simulink model "Dynamics"  (R2025b)
settings: Solver=VariableStepAuto  StartTime=0.0  StopTime=400000000.0  RelTol=1e-3
values from neighbouring files (symbols this model uses):
  Jc = [400, 0, 0 ... (first row only)    [model.m]
  Jc1 = inv(Jc)    [model.m]
  mu = 3.986004418e14    (= 398600441800000)    [model.m]
  r = 1e6    (= 1000000)    [model.m]
libraries: matrix_library x2, dspmathops x1
settings Model: Creator=sstef  LastModifiedBy=sstef

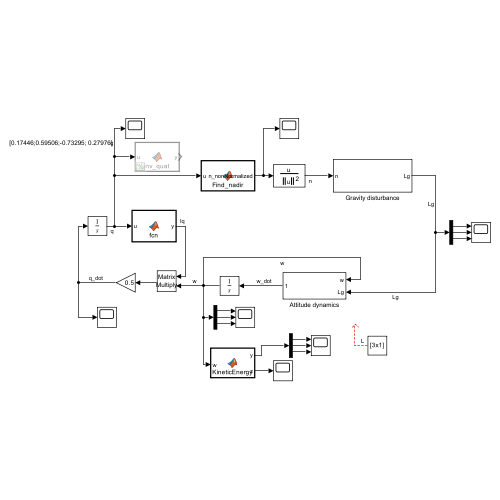
[thumbnail: Simulink's stored preview of the top-level diagram]
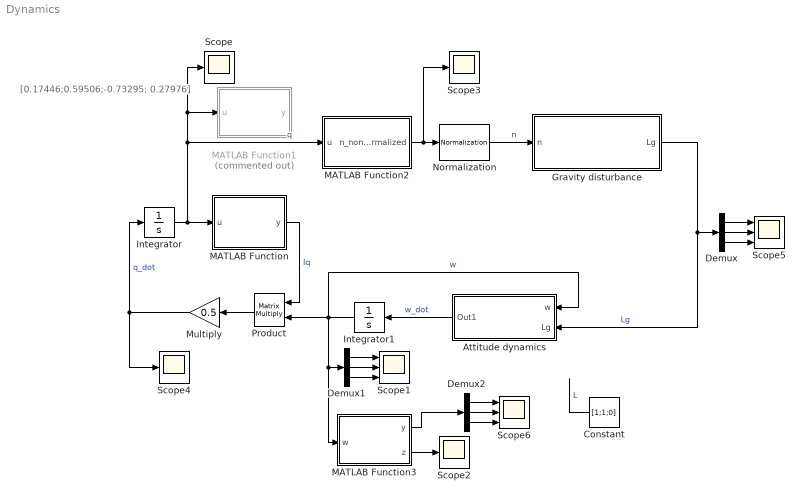
== system Dynamics ==
  note: [0.17446;0.59506;-0.73295; 0.27976]
  Attitude dynamics : Subsystem
  Constant : Constant  Value=[1;1;0]
  Demux : Demux  Outputs=3
  Demux1 : Demux  Outputs=3
  Demux2 : Demux  Outputs=3
  Gravity disturbance : Subsystem
  Integrator : Integrator  InitialCondition=[0.17446;0.59506;-0.73295; 0.27976]  AbsoluteTolerance=0.0001
  Integrator1 : Integrator  AbsoluteTolerance=0.000001
  MATLAB Function : MATLAB Function  TreatAsAtomicUnit=on
  MATLAB Function1 : MATLAB Function  Commented=on  TreatAsAtomicUnit=on
  MATLAB Function2 : MATLAB Function  TreatAsAtomicUnit=on
  MATLAB Function3 : MATLAB Function  TreatAsAtomicUnit=on
  Multiply : Gain  Gain=0.5
  Normalization : dspmathops/Normalization  NormType=Squared 2-norm  Bias=1e-10  NormOver=Each column  Dimension=1  roundingMode=Floor  overflowMode=off  accumDataTypeStr=Inherit: Same as product output  accumLastDataTypeStr=Inherit: Same as product output  outputDataTypeStr=Inherit: Same as product output  outputMin=[]  outputMax=[]  outputLastDataTypeStr=Inherit: Same as product output
  Product : Product  Multiplication=Matrix(*)
  Scope{,2..4} (4 alike) : Scope
      Scope settings: ActiveDisplayYMinimum=-1.1073586484383933  ActiveDisplayYMaximum=1.0833772002903839
      Scope2 settings: ActiveDisplayYMinimum=-0.0045801648053489111  ActiveDisplayYMaximum=0.041221483248140206  DataLoggingVariableName=ScopeData2
      Scope3 settings: ActiveDisplayYMinimum=-1.0201256866840489  ActiveDisplayYMaximum=1.2244583915622078  DataLoggingVariableName=ScopeData6
      Scope4 settings: ActiveDisplayYMinimum=-1.7498948486538512E+34  ActiveDisplayYMaximum=1.6554770346850636E+34  DataLoggingVariableName=ScopeData7
  Scope1 : Scope  NumInputPorts=3
      settings: ActiveDisplayYMinimum=-0.0069359480951209015  ActiveDisplayYMaximum=0.0069181215637571323
  Scope5 : Scope  NumInputPorts=3
      settings: ActiveDisplayYMinimum=-0.013350016010267451  ActiveDisplayYMaximum=0.013181324777865785  DataLoggingVariableName=ScopeData8
  Scope6 : Scope  NumInputPorts=3
      settings: ActiveDisplayYMinimum=-3.5092099871581417  ActiveDisplayYMaximum=3.5511518209448742  DataLoggingVariableName=ScopeData9
  wires:
  Integrator/1 -> MATLAB Function2/1(u), Scope/1, MATLAB Function1/1(u), MATLAB Function/1(u)  "q"
  Product/1 -> Multiply/1
  MATLAB Function/1(y) -> Product/1  "Iq"
  Multiply/1 -> Integrator/1, Scope4/1  "q_dot"
  Integrator1/1 -> Product/2, MATLAB Function3/1(w), Demux1/1, Attitude dynamics/1(w)  "w"
  Attitude dynamics/1(Out1) -> Integrator1/1  "w_dot"
  Constant/1 -> ?  "L"
  MATLAB Function2/1(n_nonNormalized) -> Scope3/1, Normalization/1
  Demux/2 -> Scope5/2
  Demux/3 -> Scope5/3
  Demux/1 -> Scope5/1
  Demux1/1 -> Scope1/1
  Demux1/3 -> Scope1/3
  Demux1/2 -> Scope1/2
  Gravity disturbance/1(Lg) -> Attitude dynamics/2(Lg), Demux/1  "Lg"
  Normalization/1 -> Gravity disturbance/1(n)  "n"
  MATLAB Function3/1(y) -> Demux2/1
  MATLAB Function3/2(z) -> Scope2/1
  Demux2/2 -> Scope6/2
  Demux2/3 -> Scope6/3
  Demux2/1 -> Scope6/1

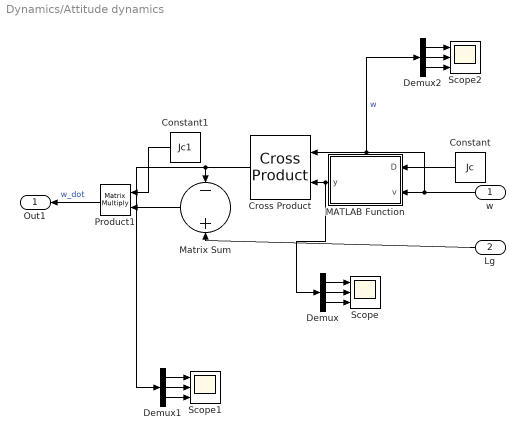
== system Dynamics/Attitude dynamics ==
  w : Inport
  Lg : Inport  Port=2
  Constant : Constant  Value=Jc
  Constant1 : Constant  Value=Jc1
  Cross Product : matrix_library/Cross Product
  Demux : Demux  Outputs=3
  Demux1 : Demux  Outputs=3
  Demux2 : Demux  Outputs=3
  MATLAB Function : MATLAB Function  TreatAsAtomicUnit=on
  Matrix Sum : Sum  Inputs=-+
  Product1 : Product  Multiplication=Matrix(*)
  Scope : Scope  NumInputPorts=3
      settings: ActiveDisplayYMinimum=-84.730783605714521  ActiveDisplayYMaximum=82.344369944838959  DataLoggingVariableName=ScopeData3
  Scope1 : Scope  NumInputPorts=3
      settings: ActiveDisplayYMinimum=-1.8791066376898631E-10  ActiveDisplayYMaximum=4.2850622121844011E-11  DataLoggingVariableName=ScopeData4
  Scope2 : Scope  NumInputPorts=3
      settings: ActiveDisplayYMinimum=-0.0027775205734021252  ActiveDisplayYMaximum=0.024997685160619131  DataLoggingVariableName=ScopeData5
  Out1 : Outport
  wires:
  w/1 -> Demux2/1, Cross Product/1, MATLAB Function/2(v)  "w"
  Lg/1 -> Matrix Sum/2
  Constant1/1 -> Product1/1
  Matrix Sum/1 -> Product1/2
  Product1/1 -> Out1/1  "w_dot"
  Constant/1 -> MATLAB Function/1(D)
  MATLAB Function/1(y) -> Demux/1, Cross Product/2
  Demux/1 -> Scope/1
  Demux/2 -> Scope/2
  Demux/3 -> Scope/3
  Demux1/2 -> Scope1/2
  Demux1/1 -> Scope1/1
  Cross Product/1 -> Demux1/1, Matrix Sum/1
  Demux1/3 -> Scope1/3
  Demux2/2 -> Scope2/2
  Demux2/1 -> Scope2/1
  Demux2/3 -> Scope2/3

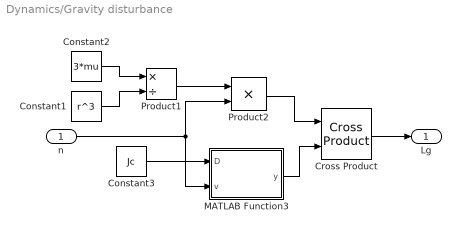
== system Dynamics/Gravity disturbance ==
  n : Inport
  Constant1 : Constant  Value=r^3
  Constant2 : Constant  Value=3*mu
  Constant3 : Constant  Value=Jc
  Cross Product : matrix_library/Cross Product
  MATLAB Function3 : MATLAB Function  TreatAsAtomicUnit=on
  Product1 : Product  Inputs=*/
  Product2 : Product
  Lg : Outport
  wires:
  Cross Product/1 -> Lg/1
  Product1/1 -> Product2/1
  n/1 -> Product2/2, MATLAB Function3/2(v)
  MATLAB Function3/1(y) -> Cross Product/2
  Constant1/1 -> Product1/2
  Constant2/1 -> Product1/1
  Constant3/1 -> MATLAB Function3/1(D)
  Product2/1 -> Cross Product/1

== matlab function Dynamics/MATLAB Function ==
  data: u input size=4 1; y output size=4 3
function y  = fcn(u)
% 
% q4=u(4);
% q_vect=u(1:3);
% qx=[0,  -q_vect(3)  q_vect(2);
%     q_vect(3), 0,  -q_vect(1);
%     -q_vect(2), q_vect(1), 0];
% 
% Iq=[diag([q4, q4, q4])+qx;
%       -q_vect.'  ];
% y = Iq;

y=[u(4), -u(3), u(2);
    u(3), u(4), -u(1);
    -u(2), u(1), u(4);
    -u(1),-u(2),-u(3);];

== matlab function Dynamics/Attitude dynamics/MATLAB Function ==
  data: D input size=[3 3]; y output size=[3 1]; v input size=[3 1]
function y = Matrix_Product(D, v)
u=diag3_vector_product(D, v);
y = u.';

== matlab function Dynamics/MATLAB Function2 ==
  data: u input; n_nonNormalized output
function n_nonNormalized = Find_nadir(u)
q_first=scalarLast_toFirst(u);
n_nonNormalized=(rotate_by_quat(q_first.',[0, 0, -1]));

== matlab function Dynamics/Gravity disturbance/MATLAB Function3 ==
  data: D input size=[3 3]; y output size=[3 1]; v input size=[3 1]
function y = Matrix_Product(D, v)
u=diag3_vector_product(D, v);
y = u.';

== matlab function Dynamics/MATLAB Function3 ==
  data: w input; y output; z output
function [y, z]= KineticEnergy(w)
Jc=[400, 0, 0;
    0, 500, 0;
    0, 0, 450;];
y=Jc*w;
z=0.5*w'*y;

== matlab function Dynamics/MATLAB Function1 ==
  data: u input; y output
function y = inv_quat(u)
q_first=scalarLast_toFirst(u);
q_invFirst=quatinv(q_first.');
q_inv=scalarFirst_toLast(q_invFirst.');
y = q_inv;
